simulink model "model_sample_nuttx"  (R2019b)
settings: Solver=FixedStepDiscrete  StartTime=0.0  StopTime=10.0  RelTol=1e-3  EnableMultiTasking=on
settings Model: SimulationMode=external  Creator=guest  LastModifiedBy=pi
settings DataIOCC: ReturnWorkspaceOutputs=off
settings OptimizationCC: EnhancedBackFolding=on  PassReuseOutputArgsAs=Individual arguments  ZeroExternalMemoryAtStartup=off  ZeroInternalMemoryAtStartup=off  OptimizeBlockOrder=speed  DifferentSizesBufferReuse=on  OptimizationCustomize=off  EfficientTunableParamExpr=on
settings DebuggingCC: ParameterTunabilityLossMsg=error  ArithmeticOperatorsInVariantConditions=warning
settings SFSimCC: SimUseLocalCustomCode=off  MATLABDynamicMemAlloc=off  CustomCodeUndefinedFunction=UseInterfaceOnly
settings RTWCC: Description=NuttX Embedded Coder  SystemTargetFile=ert_nuttx.tlc  MakeCommand=make_rtw NUTTX_EXPORT=/path/to/nuttx-export  TemplateMakefile=ert_nuttx.tmf  GenerateReport=on  RTWUseLocalCustomCode=off  IncludeHyperlinkInReport=on  LaunchReport=on  GenerateTraceInfo=on  GenerateTraceReport=on  GenerateTraceReportSl=on  GenerateTraceReportSf=on  GenerateTraceReportEml=on
settings CodeAppCC: ForceParamTrailComments=on  IgnoreCustomStorageClasses=off  OperatorAnnotations=on  SimulinkDataObjDesc=on  SFDataObjDesc=on  MATLABFcnDesc=on  InsertBlockDesc=on
settings STFCustomTargetCC: TargetLangStandard=C99 (ISO)  MultiwordLength=256  ModelReferenceCompliant=off  CombineOutputUpdateFcns=on  ERTCustomFileBanners=on  SupportContinuousTime=off  RemoveResetFunc=on  MATLABClassNameForMDSCustomization=Simulink.SoftwareTarget.ERTCustomization  SystemTargetFile=ert_nuttx.tlc
settings ERTTargetCC: TargetLangStandard=C99 (ISO)  ModelReferenceCompliant=off  ParMdlRefBuildCompliant=off  CompOptLevelCompliant=off  ConcurrentExecutionCompliant=off  SupportNonInlinedSFcns=on  ModelStepFunctionPrototypeControlCompliant=off  CPPClassGenCompliant=off  UseToolchainInfoCompliant=off  ExtMode=on  ExtModeMexArgs='192.168.1.43'  ERTCustomFileTemplate=ert_linux_file_process.tlc

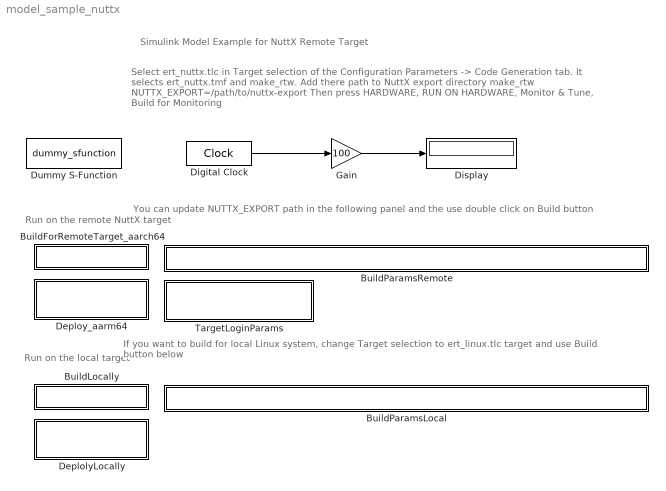
== system model_sample_nuttx ==
  note: You can update NUTTX_EXPORT path in the following panel and the use double click on Build button
  note: Select ert_nuttx.tlc in Target selection of the Configuration Parameters -> Code Generation tab.
      | It selects  ert_nuttx.tmf and make_rtw. Add there path to NuttX export directory
      | make_rtw NUTTX_EXPORT=/path/to/nuttx-export
      | Then press HARDWARE, RUN ON HARDWARE, Monitor & Tune, Build for Monitoring
  note: Simulink Model Example for NuttX Remote Target
  note: Run on the local target
  note: Run on the remote NuttX target
  note: If you want to build for local Linux system, change Target selection to ert_linux.tlc target and use Build button below
  BuildForRemoteTarget_aarch64 : Subsystem
      settings: OpenFcn=ert_linux_build(gcs, 'BuildParamsRemote');
      mask Display: disp('Build')
  BuildLocally : Subsystem
      settings: OpenFcn=ert_linux_build(gcs, 'BuildParamsLocal');
      mask Display: disp('Build')
  BuildParamsLocal : Subsystem  mask{make_command='make_rtw OPT_OPTS="-O2 -ggdb -Wall" CC=gcc'}
      mask prompts: make_command "MakeCommand"
      mask Display: disp(get_param(gcb, 'make_command'));
  BuildParamsRemote : Subsystem  mask{make_command='make_rtw NUTTX_EXPORT=/path/to/nuttx-export'}
      mask prompts: make_command "MakeCommand"
      mask Display: disp(get_param(gcb, 'make_command'));
  DeplolyLocally : Subsystem
      settings: OpenFcn=ert_linux_deploy_and_connect(gcs);
      mask Display: disp('Deploy and\nconnect')
  Deploy_aarm64 : Subsystem
      settings: OpenFcn=ert_linux_deploy_and_connect(gcs, 'TargetLoginParams');
      mask Display: disp('Deploy and\nconnect')
  Digital Clock : DigitalClock
  Display : Display
  Dummy S-Function : S-Function  FunctionName=dummy_sfunction  Parameters=-1  SFunctionDeploymentMode=off  EnableBusSupport=off
  Gain : Gain  Gain=100
  TargetLoginParams : Subsystem  mask{trgt_ip_addr='192.168.1.43', trgt_username='user'}
      mask prompts: trgt_ip_addr "Target IP address"; trgt_username "Target username"
      mask Display:
      | ip_addr = get_param(gcb, 'trgt_ip_addr');
      | user = get_param(gcb, 'trgt_username');
      | 
      | fprintf('IP addr:\t %s\n User:\t %s ', ip_addr, user);
  wires:
  Digital Clock/1 -> Gain/1
  Gain/1 -> Display/1

== system model_sample_nuttx/BuildForRemoteTarget_aarch64 ==

== system model_sample_nuttx/BuildLocally ==

== system model_sample_nuttx/BuildParamsLocal ==

== system model_sample_nuttx/BuildParamsRemote ==

== system model_sample_nuttx/DeplolyLocally ==

== system model_sample_nuttx/Deploy_aarm64 ==

== system model_sample_nuttx/TargetLoginParams ==
